simulink model "axi_filter_KCM_RC_EV"  (R2020a)
settings: Solver=VariableStepAuto  StartTime=0.0  StopTime=(height*width)/fs + (width*6)/fs + 128/fs  RelTol=1e-3
PreLoadFcn:
  | clear all;
  | 
  | fs = 100e6;
PostLoadFcn:
  | ratio = 1/6;
  | set(0,'units','pixels');
  | pixels = get(0,'screensize');
  | point1 = round(pixels(3)*ratio);
  | point2 = round(pixels(4)*ratio);
  | point3 = pixels(3)-round(pixels(3)*ratio);
  | point4 = pixels(4)-round(pixels(4)*ratio);
  | h = get_param(gcs,'handle');
  | set_param(h,'location',[point1 point2 point3 point4]);
  | pause(0.2);
  | set_param(h,'Zoomfactor','fit to view');
  | 
  | clear ratio pixels point1 point2 point3 point4 h
  | 
  | % https://uk.mathworks.com/matlabcentral/answers/358413-open-simulink-model-with-set-window-size-and-position
InitFcn:
  | height = str2num(get_param([bdroot, '/Image Properties'], 'height'));
  | width = str2num(get_param([bdroot, '/Image Properties'], 'width'));
  | I = imresize(eval(get_param([bdroot, '/Image Properties'], 'image')), [(height) (width)]);
  | I = padarray(I, [1 1], 'replicate');
  | bufferOut = uint32(double(I(:,:,1))*2^16 + double(I(:,:,3))*2^8 + double(I(:,:,2)));
  | bufferOut = reshape(bufferOut', [width+2, height+2]);
  | bufferOut = bufferOut(:);
StopFcn:
  | imtool(I);
  | imtool(uint8(reshape(bufferIn, [width, height])'));
undefined symbols (not defined in the file): AXI4, Lite
libraries: xbsIndex_r4 x114, hdlsllib x3, dspsrcs4 x2, simulink x1
(part 1 of 2)
settings Model: Creator=David Northcote  LastModifiedBy=qhb21126
settings DataIOCC: ReturnWorkspaceOutputs=off
settings DebuggingCC: ArithmeticOperatorsInVariantConditions=warning
settings SFSimCC: SimUseLocalCustomCode=off  CustomCodeUndefinedFunction=UseInterfaceOnly
settings RTWCC: RTWUseLocalCustomCode=off

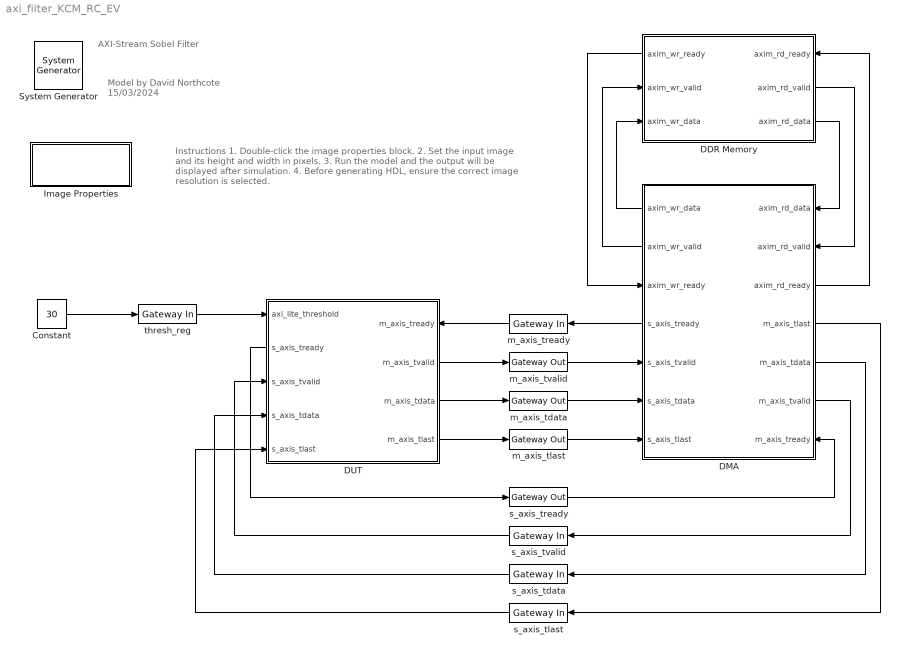
== system axi_filter_KCM_RC_EV ==
  note: Instructions
      |
      | 1. Double-click the image properties block.
      |
      | 2. Set the input image and its height and width in pixels.
      |
      | 3. Run the model and the output will be displayed after simulation.
      |
      | 4. Before generating HDL, ensure the correct image resolution is selected.
  note: Model by David Northcote
      | 15/03/2024
  note: AXI-Stream Sobel Filter
  " System Generator" : xbsIndex_r4/ System Generator  Tag=genX  xilinxfamily=zynq  part=xc7z020  speed=-1  package=clg400  synthesis_tool=Vivado  clock_wrapper=Clock Enables  directory=./netlist  proj_type=Vivado  Synth_file=Vivado Synthesis Defaults  Impl_file=Vivado Implementation Defaults  testbench=off  simulink_period=1/100e6  sysclk_period=10  dcm_input_clock_period=10  incr_netlist=off  trim_vbits=Everywhere in SubSystem  dbl_ovrd=According to Block Masks  core_generation=According to Block Masks  run_coregen=off  deprecated_control=off  eval_field=0  block_type=sysgen
  Constant : Constant  Value=30  SampleTime=-1
  DDR Memory : Subsystem  mask{bufferOut=bufferOut, dtype=uint32, outVar="bufferIn"}
      mask prompts: bufferOut "Data to be sent:"; dtype "Data type:"; outVar "Output variable name:"
      mask init:
      | dtypeStr = get_param(gcb, 'dtype');
      | outVarStr = get_param(gcb, 'outVar');
      | set_param([gcb, '/Buffer In/To Workspace'], 'VariableName', outVar)
      settings: PortSchema="{\"entries\":[{\"content\":{\"sides\":[{\"content\":{\"connectorIds\":[\"Out3\",\"In1\",\"In2\"]},\"type\":\"ConnectorPlacement.EquallySpacedRectSide\",\"uuid\":\"10820561-fcd3-42da-ac38-14c6f993f770\"},{\"content\":{\"connectorIds\":[\"In3\",\"Out1\",\"Out2\"],\"side\":\"RIGHT\"},\"type\":\"ConnectorPlacement.EquallySpacedRectSide\",\"uuid\":\"072276f7-1cf8-495f-bb0a-1bca7e8326ea\"},{\"content\":{\"connectorIds\":[],\"side\":\"TOP\"},\"type\":\"ConnectorPlacement.EquallySpacedRectSide\",\"uuid\":\"f5b81d71-f8e7-451c-95ca-ef44dafc9f7a\"}]},\"type\":\"ConnectorPlacement.EquallySpacedConnector\",\"uuid\":\"59ea238c-ea64-4381-b9ec-a479227d5ff5\"}],\"packageUris\":[\"http://schema.mathworks.com/mf0/Connector/19700101\"],\"version\":\"1.0\"}"
      mask TypeOptions dtype: uint32 | int32
      mask DialogControl DescGroupVar Prompt: DDR Memory
      mask DialogControl DescTextVar Prompt: Block simulating a DDR memory controller.
      mask DialogControl ParameterGroupVar Prompt: MM2S
      mask DialogControl Container4 Prompt: S2MM
  DMA : Subsystem  mask{N=length(bufferOut(:))}
      mask prompts: N "Length of data:"
      settings: PortSchema="{\"entries\":[{\"content\":{\"sides\":[{\"content\":{\"connectorIds\":[\"Out5\",\"Out6\",\"In1\",\"Out7\",\"In2\",\"In3\",\"In4\"]},\"type\":\"ConnectorPlacement.EquallySpacedRectSide\",\"uuid\":\"c102abcb-2e00-4fd7-85df-5b9b0b898bd0\"},{\"content\":{\"connectorIds\":[\"In5\",\"In6\",\"Out1\",\"Out2\",\"Out3\",\"Out4\",\"In7\"],\"side\":\"RIGHT\"},\"type\":\"ConnectorPlacement.EquallySpacedRectSide\",\"uuid\":\"9e178eef-1e1d-41e3-971e-2eb7c6a5387e\"},{\"content\":{\"connectorIds\":[],\"side\":\"TOP\"},\"type\":\"ConnectorPlacement.EquallySpacedRectSide\",\"uuid\":\"12cf59e0-f07a-41d8-b174-5a1eb72b1624\"},{\"content\":{\"connectorIds\":[],\"side\":\"BOTTOM\"},\"type\":\"ConnectorPlacement.EquallySpacedRectSide\",\"uuid\":\"a47cc6bb-72ec-4c9c-b625-c22428f6e2e0\"}]},\"type\":\"ConnectorPlacement.EquallySpacedConnector\",\"uuid\":\"cad21ed4-9065-49eb-a891-849a058d114a\"}],\"packageUris\":[\"http://schema.mathworks.com/mf0/Connector/19700101\"],\"version\":\"1.0\"}"
      mask DialogControl DescGroupVar Prompt: AXI DMA
      mask DialogControl DescTextVar Prompt: Block simulating an AXI DMA.
      mask DialogControl ParameterGroupVar Prompt: Main
  DUT : Subsystem
      settings: PortSchema="{\"entries\":[{\"content\":{\"sides\":[{\"content\":{\"connectorIds\":[\"In1\",\"Out4\",\"In2\",\"In3\",\"In4\"]},\"type\":\"ConnectorPlacement.EquallySpacedRectSide\",\"uuid\":\"c102abcb-2e00-4fd7-85df-5b9b0b898bd0\"},{\"content\":{\"connectorIds\":[\"In5\",\"Out1\",\"Out2\",\"Out3\"],\"side\":\"RIGHT\"},\"type\":\"ConnectorPlacement.EquallySpacedRectSide\",\"uuid\":\"9e178eef-1e1d-41e3-971e-2eb7c6a5387e\"},{\"content\":{\"connectorIds\":[],\"side\":\"TOP\"},\"type\":\"ConnectorPlacement.EquallySpacedRectSide\",\"uuid\":\"12cf59e0-f07a-41d8-b174-5a1eb72b1624\"}]},\"type\":\"ConnectorPlacement.EquallySpacedConnector\",\"uuid\":\"cad21ed4-9065-49eb-a891-849a058d114a\"}],\"packageUris\":[\"http://schema.mathworks.com/mf0/Connector/19700101\"],\"version\":\"1.0\"}"
  Image Properties : Subsystem  mask{image=imread('Louise.png'), height=317, width=313}
      mask prompts: image "Input Image:"; height "Image Height:"; width "Image Width:"
      mask init:
      | str = [width];
      mask DialogControl DescGroupVar Prompt: Image Properties
      mask DialogControl DescTextVar Prompt: Set the image and its size using the parameters below.
      mask DialogControl ParameterGroupVar Prompt: Main
      mask Display: disp('Properties')
  m_axis_tdata : xbsIndex_r4/Gateway Out  inherit_from_input=on  hdl_port=on  rows=1  columns=1  UseAsDAC=off  DACChannel='1'  interface=None  automatic_assignment=on  address_offset=hex2dec('00')  intf_name=''  intf_description=''  timing_constraint=None  locs_specified=off  LOCs={}  io_standard={}  block_type=gatewayout
  m_axis_tlast : xbsIndex_r4/Gateway Out  inherit_from_input=on  hdl_port=on  rows=1  columns=1  UseAsDAC=off  DACChannel='1'  interface=None  automatic_assignment=on  address_offset=hex2dec('00')  intf_name=''  intf_description=''  timing_constraint=None  locs_specified=off  LOCs={}  io_standard={}  block_type=gatewayout
  m_axis_tready : xbsIndex_r4/Gateway In  gui_display_data_type=Boolean  arith_type=Boolean  n_bits=16  bin_pt=14  preci_type=Single  exp_width=8  frac_width=24  rows=1  columns=1  quantization="Round  (unbiased: +/- Inf)"  overflow=Saturate  period=1/fs  UseAsADC=off  ADCChannel='1'  interface=None  automatic_assignment=on  address_offset=hex2dec('00')  intf_name=''  intf_description=''  default_value=0  timing_constraint=None  locs_specified=off  LOCs={}  io_standard={}  inherit_from_input=off  hdl_port=on  dbl_ovrd=off  block_type=gatewayin
  m_axis_tvalid : xbsIndex_r4/Gateway Out  inherit_from_input=on  hdl_port=on  rows=1  columns=1  UseAsDAC=off  DACChannel='1'  interface=None  automatic_assignment=on  address_offset=hex2dec('00')  intf_name=''  intf_description=''  timing_constraint=None  locs_specified=off  LOCs={}  io_standard={}  block_type=gatewayout
  s_axis_tdata : xbsIndex_r4/Gateway In  gui_display_data_type=Fixed-point  arith_type=Unsigned  n_bits=32  bin_pt=0  preci_type=Single  exp_width=8  frac_width=24  rows=1  columns=1  quantization="Round  (unbiased: +/- Inf)"  overflow=Saturate  period=1/fs  UseAsADC=off  ADCChannel='1'  interface=None  automatic_assignment=on  address_offset=hex2dec('00')  intf_name=''  intf_description=''  default_value=0  timing_constraint=None  locs_specified=off  LOCs={}  io_standard={}  inherit_from_input=off  hdl_port=on  dbl_ovrd=off  block_type=gatewayin
  s_axis_tlast : xbsIndex_r4/Gateway In  gui_display_data_type=Boolean  arith_type=Boolean  n_bits=16  bin_pt=14  preci_type=Single  exp_width=8  frac_width=24  rows=1  columns=1  quantization="Round  (unbiased: +/- Inf)"  overflow=Saturate  period=1/fs  UseAsADC=off  ADCChannel='1'  interface=None  automatic_assignment=on  address_offset=hex2dec('00')  intf_name=''  intf_description=''  default_value=0  timing_constraint=None  locs_specified=off  LOCs={}  io_standard={}  inherit_from_input=off  hdl_port=on  dbl_ovrd=off  block_type=gatewayin
  s_axis_tready : xbsIndex_r4/Gateway Out  inherit_from_input=on  hdl_port=on  rows=1  columns=1  UseAsDAC=off  DACChannel='1'  interface=None  automatic_assignment=on  address_offset=hex2dec('00')  intf_name=''  intf_description=''  timing_constraint=None  locs_specified=off  LOCs={}  io_standard={}  block_type=gatewayout
  s_axis_tvalid : xbsIndex_r4/Gateway In  gui_display_data_type=Boolean  arith_type=Boolean  n_bits=16  bin_pt=14  preci_type=Single  exp_width=8  frac_width=24  rows=1  columns=1  quantization="Round  (unbiased: +/- Inf)"  overflow=Saturate  period=1/fs  UseAsADC=off  ADCChannel='1'  interface=None  automatic_assignment=on  address_offset=hex2dec('00')  intf_name=''  intf_description=''  default_value=0  timing_constraint=None  locs_specified=off  LOCs={}  io_standard={}  inherit_from_input=off  hdl_port=on  dbl_ovrd=off  block_type=gatewayin
  thresh_reg : xbsIndex_r4/Gateway In  gui_display_data_type=Fixed-point  arith_type=Unsigned  n_bits=32  bin_pt=0  preci_type=Single  exp_width=8  frac_width=24  rows=1  columns=1  quantization="Round  (unbiased: +/- Inf)"  overflow=Saturate  period=1/fs  UseAsADC=off  ADCChannel='1'  interface=AXI4-Lite  automatic_assignment=on  address_offset=hex2dec('00')  intf_name=''  intf_description=''  default_value=0  timing_constraint=None  locs_specified=off  LOCs={}  io_standard={}  inherit_from_input=off  hdl_port=on  dbl_ovrd=off  block_type=gatewayin
  wires:
  s_axis_tvalid/1 -> DUT/2(s_axis_tvalid)
  s_axis_tdata/1 -> DUT/3(s_axis_tdata)
  s_axis_tlast/1 -> DUT/4(s_axis_tlast)
  m_axis_tready/1 -> DUT/5(m_axis_tready)
  DUT/4(s_axis_tready) -> s_axis_tready/1
  DUT/2(m_axis_tdata) -> m_axis_tdata/1
  DUT/1(m_axis_tvalid) -> m_axis_tvalid/1
  DUT/3(m_axis_tlast) -> m_axis_tlast/1
  s_axis_tready/1 -> DMA/7(m_axis_tready)
  DMA/4(m_axis_tvalid) -> s_axis_tvalid/1
  DMA/3(m_axis_tdata) -> s_axis_tdata/1
  DMA/2(m_axis_tlast) -> s_axis_tlast/1
  DMA/7(s_axis_tready) -> m_axis_tready/1
  m_axis_tvalid/1 -> DMA/2(s_axis_tvalid)
  m_axis_tdata/1 -> DMA/3(s_axis_tdata)
  m_axis_tlast/1 -> DMA/4(s_axis_tlast)
  DMA/1(axim_rd_ready) -> DDR Memory/3(axim_rd_ready)
  DDR Memory/1(axim_rd_valid) -> DMA/6(axim_rd_valid)
  DDR Memory/2(axim_rd_data) -> DMA/5(axim_rd_data)
  DDR Memory/3(axim_wr_ready) -> DMA/1(axim_wr_ready)
  DMA/6(axim_wr_valid) -> DDR Memory/1(axim_wr_valid)
  DMA/5(axim_wr_data) -> DDR Memory/2(axim_wr_data)
  thresh_reg/1 -> DUT/1(axi_lite_threshold)
  Constant/1 -> thresh_reg/1

== system axi_filter_KCM_RC_EV/DDR Memory ==
  axim_wr_valid : Inport
  axim_wr_data : Inport  Port=2
  axim_rd_ready : Inport  Port=3
  AXI Read Scope : Scope  NumInputPorts=3
  AXI Write Scope : Scope  NumInputPorts=3
  Buffer In : Subsystem
  Buffer Out : Subsystem
  axim_rd_valid : Outport
  axim_rd_data : Outport  Port=2
  axim_wr_ready : Outport  Port=3
  wires:
  Buffer Out/1(Valid) -> AXI Read Scope/1, axim_rd_valid/1
  Buffer Out/2(Data) -> AXI Read Scope/2, axim_rd_data/1
  axim_rd_ready/1 -> Buffer Out/Enable, AXI Read Scope/3
  axim_wr_data/1 -> AXI Write Scope/2, Buffer In/1(Data)
  Buffer In/1(Ready) -> AXI Write Scope/3, axim_wr_ready/1
  axim_wr_valid/1 -> Buffer In/Enable, AXI Write Scope/1

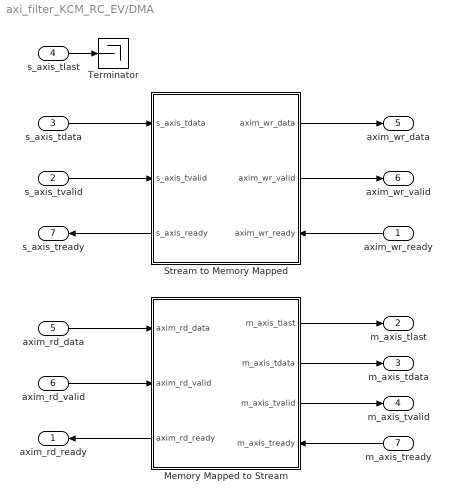
== system axi_filter_KCM_RC_EV/DMA ==
  axim_wr_ready : Inport
  s_axis_tvalid : Inport  Port=2
  s_axis_tdata : Inport  Port=3
  s_axis_tlast : Inport  Port=4
  axim_rd_data : Inport  Port=5
  axim_rd_valid : Inport  Port=6
  m_axis_tready : Inport  Port=7
  Memory Mapped to Stream : Subsystem
      settings: PortSchema="{\"entries\":[{\"content\":{\"sides\":[{\"content\":{\"connectorIds\":[\"In1\",\"In2\",\"Out4\"]},\"type\":\"ConnectorPlacement.EquallySpacedRectSide\",\"uuid\":\"10820561-fcd3-42da-ac38-14c6f993f770\"},{\"content\":{\"connectorIds\":[\"Out1\",\"Out2\",\"Out3\",\"In3\"],\"side\":\"RIGHT\"},\"type\":\"ConnectorPlacement.EquallySpacedRectSide\",\"uuid\":\"072276f7-1cf8-495f-bb0a-1bca7e8326ea\"},{\"content\":{\"connectorIds\":[],\"side\":\"TOP\"},\"type\":\"ConnectorPlacement.EquallySpacedRectSide\",\"uuid\":\"f5b81d71-f8e7-451c-95ca-ef44dafc9f7a\"}]},\"type\":\"ConnectorPlacement.EquallySpacedConnector\",\"uuid\":\"59ea238c-ea64-4381-b9ec-a479227d5ff5\"}],\"packageUris\":[\"http://schema.mathworks.com/mf0/Connector/19700101\"],\"version\":\"1.0\"}"
  Stream to Memory Mapped : Subsystem
      settings: PortSchema="{\"entries\":[{\"content\":{\"sides\":[{\"content\":{\"connectorIds\":[\"In1\",\"In2\",\"Out3\"]},\"type\":\"ConnectorPlacement.EquallySpacedRectSide\",\"uuid\":\"10820561-fcd3-42da-ac38-14c6f993f770\"},{\"content\":{\"connectorIds\":[\"Out1\",\"Out2\",\"In3\"],\"side\":\"RIGHT\"},\"type\":\"ConnectorPlacement.EquallySpacedRectSide\",\"uuid\":\"072276f7-1cf8-495f-bb0a-1bca7e8326ea\"},{\"content\":{\"connectorIds\":[],\"side\":\"TOP\"},\"type\":\"ConnectorPlacement.EquallySpacedRectSide\",\"uuid\":\"f5b81d71-f8e7-451c-95ca-ef44dafc9f7a\"}]},\"type\":\"ConnectorPlacement.EquallySpacedConnector\",\"uuid\":\"59ea238c-ea64-4381-b9ec-a479227d5ff5\"}],\"packageUris\":[\"http://schema.mathworks.com/mf0/Connector/19700101\"],\"version\":\"1.0\"}"
  Terminator : Terminator
  axim_rd_ready : Outport
  m_axis_tlast : Outport  Port=2  VectorParamsAs1DForOutWhenUnconnected=off
  m_axis_tdata : Outport  Port=3  VectorParamsAs1DForOutWhenUnconnected=off
  m_axis_tvalid : Outport  Port=4  VectorParamsAs1DForOutWhenUnconnected=off
  axim_wr_data : Outport  Port=5
  axim_wr_valid : Outport  Port=6
  s_axis_tready : Outport  Port=7  VectorParamsAs1DForOutWhenUnconnected=off
  wires:
  m_axis_tready/1 -> Memory Mapped to Stream/3(m_axis_tready)
  Memory Mapped to Stream/1(m_axis_tlast) -> m_axis_tlast/1
  Memory Mapped to Stream/2(m_axis_tdata) -> m_axis_tdata/1
  Memory Mapped to Stream/3(m_axis_tvalid) -> m_axis_tvalid/1
  s_axis_tvalid/1 -> Stream to Memory Mapped/2(s_axis_tvalid)
  s_axis_tdata/1 -> Stream to Memory Mapped/1(s_axis_tdata)
  Stream to Memory Mapped/3(s_axis_ready) -> s_axis_tready/1
  s_axis_tlast/1 -> Terminator/1
  Stream to Memory Mapped/1(axim_wr_data) -> axim_wr_data/1
  Stream to Memory Mapped/2(axim_wr_valid) -> axim_wr_valid/1
  axim_wr_ready/1 -> Stream to Memory Mapped/3(axim_wr_ready)
  Memory Mapped to Stream/4(axim_rd_ready) -> axim_rd_ready/1
  axim_rd_data/1 -> Memory Mapped to Stream/1(axim_rd_data)
  axim_rd_valid/1 -> Memory Mapped to Stream/2(axim_rd_valid)

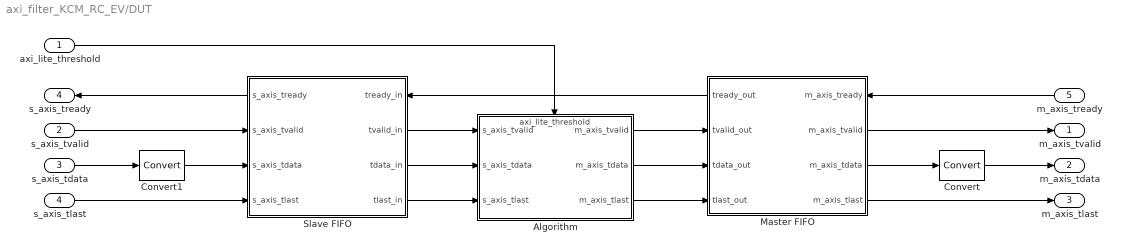
== system axi_filter_KCM_RC_EV/DUT ==
  axi_lite_threshold : Inport
  s_axis_tvalid : Inport  Port=2
  s_axis_tdata : Inport  Port=3
  s_axis_tlast : Inport  Port=4
  m_axis_tready : Inport  Port=5
  Algorithm : Subsystem
      settings: PortSchema="{\"entries\":[{\"content\":{\"sides\":[{\"content\":{\"connectorIds\":[\"In1\",\"In2\",\"In3\"]},\"type\":\"ConnectorPlacement.EquallySpacedRectSide\",\"uuid\":\"bc8f8d6b-03d4-4b1c-a4ca-076773aa8b9e\"},{\"content\":{\"connectorIds\":[\"Out1\",\"Out2\",\"Out3\"],\"side\":\"RIGHT\"},\"type\":\"ConnectorPlacement.EquallySpacedRectSide\",\"uuid\":\"0d37fd61-55f1-43d8-b642-e7957f527b3a\"},{\"content\":{\"connectorIds\":[\"In4\"],\"side\":\"TOP\"},\"type\":\"ConnectorPlacement.EquallySpacedRectSide\",\"uuid\":\"2582d54b-a3da-419d-87cd-78cc4f4daabc\"}]},\"type\":\"ConnectorPlacement.EquallySpacedConnector\",\"uuid\":\"334f8144-ee83-44bd-9d61-fffb11229a90\"}],\"packageUris\":[\"http://schema.mathworks.com/mf0/Connector/19700101\"],\"version\":\"1.0\"}"
  Convert : xbsIndex_r4/Convert  gui_display_data_type=Fixed-point  arith_type=Unsigned  n_bits=32  bin_pt=0  float_type=Single  exp_bits=8  fraction_bits=24  quantization=Truncate  overflow=Wrap  en=off  latency=0  pipeline=off  dbl_ovrd=off  block_type=convert
  Convert1 : xbsIndex_r4/Convert  gui_display_data_type=Fixed-point  arith_type=Unsigned  n_bits=24  bin_pt=0  float_type=Single  exp_bits=8  fraction_bits=24  quantization=Truncate  overflow=Wrap  en=off  latency=0  pipeline=off  dbl_ovrd=off  block_type=convert
  Master FIFO : Subsystem
      settings: PortSchema="{\"entries\":[{\"content\":{\"sides\":[{\"content\":{\"connectorIds\":[\"Out4\",\"In1\",\"In2\",\"In3\"]},\"type\":\"ConnectorPlacement.EquallySpacedRectSide\",\"uuid\":\"10820561-fcd3-42da-ac38-14c6f993f770\"},{\"content\":{\"connectorIds\":[\"In4\",\"Out1\",\"Out2\",\"Out3\"],\"side\":\"RIGHT\"},\"type\":\"ConnectorPlacement.EquallySpacedRectSide\",\"uuid\":\"072276f7-1cf8-495f-bb0a-1bca7e8326ea\"},{\"content\":{\"connectorIds\":[],\"side\":\"TOP\"},\"type\":\"ConnectorPlacement.EquallySpacedRectSide\",\"uuid\":\"f5b81d71-f8e7-451c-95ca-ef44dafc9f7a\"}]},\"type\":\"ConnectorPlacement.EquallySpacedConnector\",\"uuid\":\"59ea238c-ea64-4381-b9ec-a479227d5ff5\"}],\"packageUris\":[\"http://schema.mathworks.com/mf0/Connector/19700101\"],\"version\":\"1.0\"}"
  Slave FIFO : Subsystem
      settings: PortSchema="{\"entries\":[{\"content\":{\"sides\":[{\"content\":{\"connectorIds\":[\"Out4\",\"In1\",\"In2\",\"In3\"]},\"type\":\"ConnectorPlacement.EquallySpacedRectSide\",\"uuid\":\"10820561-fcd3-42da-ac38-14c6f993f770\"},{\"content\":{\"connectorIds\":[\"In4\",\"Out1\",\"Out2\",\"Out3\"],\"side\":\"RIGHT\"},\"type\":\"ConnectorPlacement.EquallySpacedRectSide\",\"uuid\":\"072276f7-1cf8-495f-bb0a-1bca7e8326ea\"},{\"content\":{\"connectorIds\":[],\"side\":\"TOP\"},\"type\":\"ConnectorPlacement.EquallySpacedRectSide\",\"uuid\":\"f5b81d71-f8e7-451c-95ca-ef44dafc9f7a\"}]},\"type\":\"ConnectorPlacement.EquallySpacedConnector\",\"uuid\":\"59ea238c-ea64-4381-b9ec-a479227d5ff5\"}],\"packageUris\":[\"http://schema.mathworks.com/mf0/Connector/19700101\"],\"version\":\"1.0\"}"
  m_axis_tvalid : Outport  VectorParamsAs1DForOutWhenUnconnected=off
  m_axis_tdata : Outport  Port=2  VectorParamsAs1DForOutWhenUnconnected=off
  m_axis_tlast : Outport  Port=3  VectorParamsAs1DForOutWhenUnconnected=off
  s_axis_tready : Outport  Port=4  VectorParamsAs1DForOutWhenUnconnected=off
  wires:
  Master FIFO/1(m_axis_tvalid) -> m_axis_tvalid/1
  Master FIFO/2(m_axis_tdata) -> Convert/1
  Master FIFO/3(m_axis_tlast) -> m_axis_tlast/1
  Algorithm/1(m_axis_tvalid) -> Master FIFO/1(tvalid_out)
  Algorithm/2(m_axis_tdata) -> Master FIFO/2(tdata_out)
  Algorithm/3(m_axis_tlast) -> Master FIFO/3(tlast_out)
  s_axis_tvalid/1 -> Slave FIFO/1(s_axis_tvalid)
  s_axis_tdata/1 -> Convert1/1
  s_axis_tlast/1 -> Slave FIFO/3(s_axis_tlast)
  Slave FIFO/1(tvalid_in) -> Algorithm/1(s_axis_tvalid)
  Slave FIFO/2(tdata_in) -> Algorithm/2(s_axis_tdata)
  Slave FIFO/3(tlast_in) -> Algorithm/3(s_axis_tlast)
  Slave FIFO/4(s_axis_tready) -> s_axis_tready/1
  m_axis_tready/1 -> Master FIFO/4(m_axis_tready)
  Master FIFO/4(tready_out) -> Slave FIFO/4(tready_in)
  axi_lite_threshold/1 -> Algorithm/4(axi_lite_threshold)
  Convert/1 -> m_axis_tdata/1
  Convert1/1 -> Slave FIFO/2(s_axis_tdata)

== system axi_filter_KCM_RC_EV/Image Properties ==

== system axi_filter_KCM_RC_EV/DDR Memory/Buffer In ==
  Data : Inport
  Enable : EnablePort
  Constant : Constant  OutDataTypeStr=boolean  SampleTime=-1
  To Workspace : ToWorkspace  VariableName=bufferIn  SampleTime=-1
  Ready : Outport
  wires:
  Data/1 -> To Workspace/1
  Constant/1 -> Ready/1

== system axi_filter_KCM_RC_EV/DDR Memory/Buffer Out ==
  Enable : EnablePort
  Data Type Conversion : DataTypeConversion  OutDataTypeStr=dtypeStr
  Data Type Conversion1 : DataTypeConversion  OutDataTypeStr=boolean
  Signal From Workspace : dspsrcs4/Signal From Workspace  X=bufferOut  Ts=1/fs  nsamps=1  OutputAfterFinalValue=Setting to zero  ignoreOrWarnInputAndFrameLengths=off  OutputFrames=off
  Valid Signal : dspsrcs4/Signal From Workspace  X=ones(1, length(bufferOut))  Ts=1/fs  nsamps=1  OutputAfterFinalValue=Setting to zero  ignoreOrWarnInputAndFrameLengths=off  OutputFrames=off
  Valid : Outport
  Data : Outport  Port=2
  wires:
  Signal From Workspace/1 -> Data Type Conversion/1
  Data Type Conversion/1 -> Data/1
  Valid Signal/1 -> Data Type Conversion1/1
  Data Type Conversion1/1 -> Valid/1

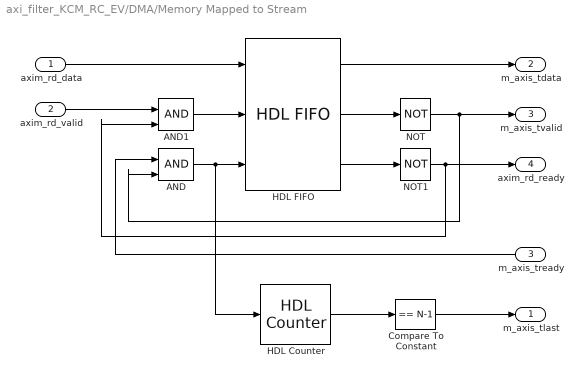
== system axi_filter_KCM_RC_EV/DMA/Memory Mapped to Stream ==
  axim_rd_data : Inport
  axim_rd_valid : Inport  Port=2
  m_axis_tready : Inport  Port=3
  AND : Logic  IconShape=distinctive  AllPortsSameDT=off  OutDataTypeStr=boolean
  AND1 : Logic  IconShape=distinctive  AllPortsSameDT=off  OutDataTypeStr=boolean
  Compare To Constant : simulink/Logic and Bit Operations/Compare To Constant  relop===  const=N-1  OutDataTypeStr=boolean
  HDL Counter : hdlsllib/Sources/HDL Counter  CountType=Count limited  CountInit=0  CountStep=1  CountMax=N-1  CountFromType=Initial value  CountFrom=0  CountResetPort=off  CountLoadPort=off  CountEnbPort=on  CountDirPort=off  CountDataType=Unsigned  CountWordLen=ceil(log2(N))  CountFracLen=0  CountSampTime=1
  HDL FIFO : hdlsllib/HDL RAMs/HDL FIFO  fifo_size=16  mode=FWFT  ratio=1  push_msg=Warning  pop_msg=Warning  show_empty=on  show_full=on  show_num=off  LabelModeActiveChoice_Mode=FWFT
      settings: SourceProductBaseCode=SL
  NOT : Logic  Operator=NOT  IconShape=distinctive  AllPortsSameDT=off  OutDataTypeStr=boolean
  NOT1 : Logic  Operator=NOT  IconShape=distinctive  AllPortsSameDT=off  OutDataTypeStr=boolean
  m_axis_tlast : Outport  VectorParamsAs1DForOutWhenUnconnected=off
  m_axis_tdata : Outport  Port=2  VectorParamsAs1DForOutWhenUnconnected=off
  m_axis_tvalid : Outport  Port=3  VectorParamsAs1DForOutWhenUnconnected=off
  axim_rd_ready : Outport  Port=4  VectorParamsAs1DForOutWhenUnconnected=off
  wires:
  NOT/1 -> m_axis_tvalid/1, AND/2
  HDL Counter/1 -> Compare To Constant/1
  m_axis_tready/1 -> AND/1
  AND/1 -> HDL Counter/1, HDL FIFO/3
  Compare To Constant/1 -> m_axis_tlast/1
  HDL FIFO/2 -> NOT/1
  AND1/1 -> HDL FIFO/2
  HDL FIFO/1 -> m_axis_tdata/1
  HDL FIFO/3 -> NOT1/1
  NOT1/1 -> AND1/2, axim_rd_ready/1
  axim_rd_valid/1 -> AND1/1
  axim_rd_data/1 -> HDL FIFO/1

== system axi_filter_KCM_RC_EV/DMA/Stream to Memory Mapped ==
  s_axis_tdata : Inport
  s_axis_tvalid : Inport  Port=2
  axim_wr_ready : Inport  Port=3
  AND : Logic  IconShape=distinctive  AllPortsSameDT=off  OutDataTypeStr=boolean
  AND1 : Logic  IconShape=distinctive  AllPortsSameDT=off  OutDataTypeStr=boolean
  HDL FIFO : hdlsllib/HDL RAMs/HDL FIFO  fifo_size=16  mode=FWFT  ratio=1  push_msg=Warning  pop_msg=Warning  show_empty=on  show_full=on  show_num=off  LabelModeActiveChoice_Mode=FWFT
      settings: SourceProductBaseCode=SL
  NOT : Logic  Operator=NOT  IconShape=distinctive  AllPortsSameDT=off  OutDataTypeStr=boolean
  NOT1 : Logic  Operator=NOT  IconShape=distinctive  AllPortsSameDT=off  OutDataTypeStr=boolean
  axim_wr_data : Outport  VectorParamsAs1DForOutWhenUnconnected=off
  axim_wr_valid : Outport  Port=2  VectorParamsAs1DForOutWhenUnconnected=off
  s_axis_ready : Outport  Port=3  VectorParamsAs1DForOutWhenUnconnected=off
  wires:
  s_axis_tvalid/1 -> AND1/1
  HDL FIFO/3 -> NOT1/1
  HDL FIFO/1 -> axim_wr_data/1
  AND1/1 -> HDL FIFO/2
  HDL FIFO/2 -> NOT/1
  AND/1 -> HDL FIFO/3
  axim_wr_ready/1 -> AND/1
  NOT/1 -> AND/2, axim_wr_valid/1
  s_axis_tdata/1 -> HDL FIFO/1
  NOT1/1 -> s_axis_ready/1, AND1/2

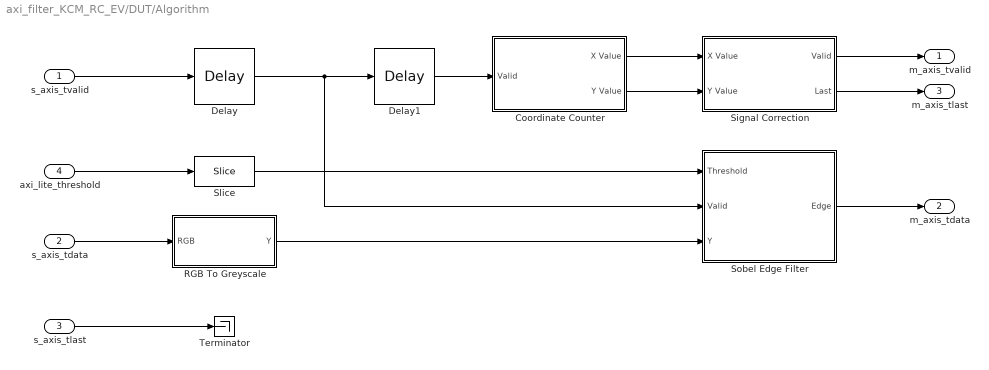
== system axi_filter_KCM_RC_EV/DUT/Algorithm ==
  s_axis_tvalid : Inport
  s_axis_tdata : Inport  Port=2
  s_axis_tlast : Inport  Port=3
  axi_lite_threshold : Inport  Port=4
  Coordinate Counter : Subsystem
  Delay : xbsIndex_r4/Delay  rst=off  infoeditControl=Selection of Reset will increase slice count due to use of real FFs and instead of SRLs  en=off  latency=3  reg_retiming=off  dbl_ovrd=off  block_type=delay
  Delay1 : xbsIndex_r4/Delay  rst=off  infoeditControl=Selection of Reset will increase slice count due to use of real FFs and instead of SRLs  en=off  latency=7  reg_retiming=off  dbl_ovrd=off  block_type=delay
  RGB To Greyscale : Subsystem
  Signal Correction : Subsystem
  Slice : xbsIndex_r4/Slice  nbits=1  boolean_output=off  mode=Two Bit Locations  bit1=7  base1=LSB of Input  bit0=0  base0=LSB of Input  dbl_ovrd=off  block_type=slice
  Sobel Edge Filter : Subsystem
  Terminator : Terminator
  m_axis_tvalid : Outport  VectorParamsAs1DForOutWhenUnconnected=off
  m_axis_tdata : Outport  Port=2  VectorParamsAs1DForOutWhenUnconnected=off
  m_axis_tlast : Outport  Port=3  VectorParamsAs1DForOutWhenUnconnected=off
  wires:
  Delay1/1 -> Coordinate Counter/1(Valid)
  Delay/1 -> Sobel Edge Filter/2(Valid), Delay1/1
  Coordinate Counter/2(Y Value) -> Signal Correction/2(Y Value)
  Coordinate Counter/1(X Value) -> Signal Correction/1(X Value)
  axi_lite_threshold/1 -> Slice/1
  s_axis_tdata/1 -> RGB To Greyscale/1(RGB)
  s_axis_tlast/1 -> Terminator/1
  s_axis_tvalid/1 -> Delay/1
  Slice/1 -> Sobel Edge Filter/1(Threshold)
  Signal Correction/2(Last) -> m_axis_tlast/1
  Signal Correction/1(Valid) -> m_axis_tvalid/1
  Sobel Edge Filter/1(Edge) -> m_axis_tdata/1
  RGB To Greyscale/1(Y) -> Sobel Edge Filter/3(Y)

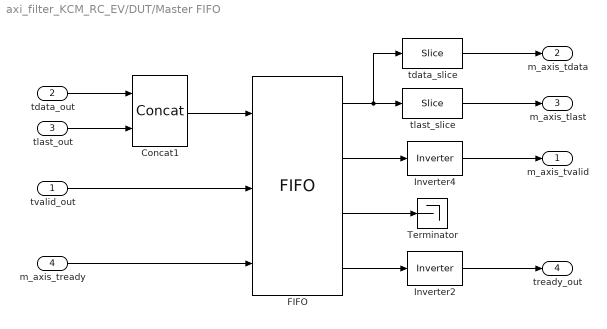
== system axi_filter_KCM_RC_EV/DUT/Master FIFO ==
  tvalid_out : Inport
  tdata_out : Inport  Port=2
  tlast_out : Inport  Port=3
  m_axis_tready : Inport  Port=4
  Concat1 : xbsIndex_r4/Concat  num_inputs=2  dbl_ovrd=off  block_type=concat
  FIFO : xbsIndex_r4/FIFO  mem_type=Block RAM  performance_options=First_Word_Fall_Through  embedded_registers=off  depth=1K  percent_nbits=1  rst=off  rst_latency=1  en=off  use_dcount=off  use_percent_full_port=off  use_almost_empty=off  almost_empty_thresh=2  use_almost_full=on  use_rd_rst_busy=off  use_wr_rst_busy=off  almost_full_thresh=1000  explicit_period=off  dbl_ovrd=off  simulation_type=fast_sim  block_type=fifo
  Inverter2 : xbsIndex_r4/Inverter  en=off  latency=0  dbl_ovrd=off  block_type=inv
  Inverter4 : xbsIndex_r4/Inverter  en=off  latency=0  dbl_ovrd=off  block_type=inv
  Terminator : Terminator
  tdata_slice : xbsIndex_r4/Slice  nbits=1  boolean_output=off  mode=Two Bit Locations  bit1=0  base1=MSB of Input  bit0=1  base0=LSB of Input  dbl_ovrd=off  block_type=slice
  tlast_slice : xbsIndex_r4/Slice  nbits=1  boolean_output=on  mode=Two Bit Locations  bit1=0  base1=LSB of Input  bit0=0  base0=LSB of Input  dbl_ovrd=off  block_type=slice
  m_axis_tvalid : Outport
  m_axis_tdata : Outport  Port=2
  m_axis_tlast : Outport  Port=3
  tready_out : Outport  Port=4
  wires:
  FIFO/4 -> Inverter2/1
  Inverter2/1 -> tready_out/1
  FIFO/2 -> Inverter4/1
  FIFO/1 -> tlast_slice/1, tdata_slice/1
  tlast_slice/1 -> m_axis_tlast/1
  tdata_slice/1 -> m_axis_tdata/1
  m_axis_tready/1 -> FIFO/3
  tvalid_out/1 -> FIFO/2
  Concat1/1 -> FIFO/1
  tdata_out/1 -> Concat1/1
  tlast_out/1 -> Concat1/2
  Inverter4/1 -> m_axis_tvalid/1
  FIFO/3 -> Terminator/1

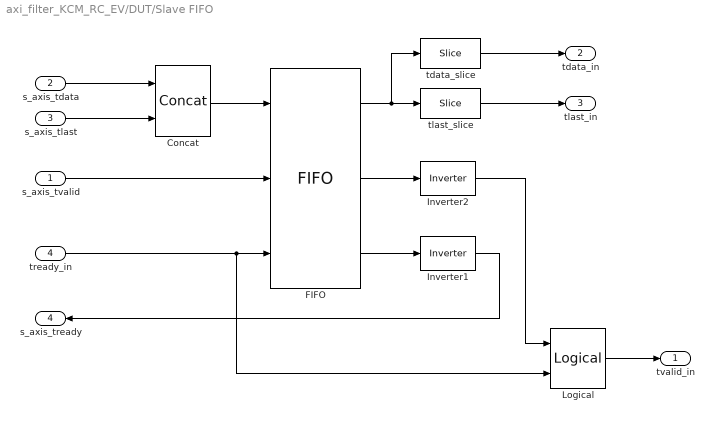
== system axi_filter_KCM_RC_EV/DUT/Slave FIFO ==
  s_axis_tvalid : Inport
  s_axis_tdata : Inport  Port=2
  s_axis_tlast : Inport  Port=3
  tready_in : Inport  Port=4
  Concat : xbsIndex_r4/Concat  num_inputs=2  dbl_ovrd=off  block_type=concat
  FIFO : xbsIndex_r4/FIFO  mem_type=Block RAM  performance_options=First_Word_Fall_Through  embedded_registers=off  depth=1K  percent_nbits=1  rst=off  rst_latency=1  en=off  use_dcount=off  use_percent_full_port=off  use_almost_empty=off  almost_empty_thresh=2  use_almost_full=off  use_rd_rst_busy=off  use_wr_rst_busy=off  almost_full_thresh=14  explicit_period=off  dbl_ovrd=off  simulation_type=fast_sim  block_type=fifo
  Inverter1 : xbsIndex_r4/Inverter  en=off  latency=0  dbl_ovrd=off  block_type=inv
  Inverter2 : xbsIndex_r4/Inverter  en=off  latency=0  dbl_ovrd=off  block_type=inv
  Logical : xbsIndex_r4/Logical  logical_function=AND  inputs=2  en=off  latency=0  precision=Full  arith_type=Unsigned  n_bits=16  bin_pt=0  align_bp=on  dbl_ovrd=off  block_type=logical
  tdata_slice : xbsIndex_r4/Slice  nbits=1  boolean_output=off  mode=Two Bit Locations  bit1=0  base1=MSB of Input  bit0=1  base0=LSB of Input  dbl_ovrd=off  block_type=slice
  tlast_slice : xbsIndex_r4/Slice  nbits=1  boolean_output=on  mode=Two Bit Locations  bit1=0  base1=LSB of Input  bit0=0  base0=LSB of Input  dbl_ovrd=off  block_type=slice
  tvalid_in : Outport
  tdata_in : Outport  Port=2
  tlast_in : Outport  Port=3
  s_axis_tready : Outport  Port=4
  wires:
  FIFO/3 -> Inverter1/1
  s_axis_tvalid/1 -> FIFO/2
  tready_in/1 -> Logical/2, FIFO/3
  Concat/1 -> FIFO/1
  s_axis_tdata/1 -> Concat/1
  s_axis_tlast/1 -> Concat/2
  FIFO/1 -> tdata_slice/1, tlast_slice/1
  tlast_slice/1 -> tlast_in/1
  tdata_slice/1 -> tdata_in/1
  Inverter1/1 -> s_axis_tready/1
  FIFO/2 -> Inverter2/1
  Inverter2/1 -> Logical/1
  Logical/1 -> tvalid_in/1

== system axi_filter_KCM_RC_EV/DUT/Algorithm/Coordinate Counter ==
  Valid : Inport
  Constant : xbsIndex_r4/Constant  const=width+1  gui_display_data_type=Fixed-point  arith_type=Unsigned  n_bits=ceil(log2(width+1))  bin_pt=0  preci_type=Single  exp_width=8  frac_width=24  explicit_period=on  period=1/100e6  equ=P=C  opselect=C  inp2=PCIN>>17  opr=+  inp1=P  carry=CIN  dbl_ovrd=off  block_type=constant
  Relational : xbsIndex_r4/Relational  mode=a=b  op_type=Bool  en=off  latency=0  dbl_ovrd=off  block_type=relational
  X Counter : xbsIndex_r4/Counter  cnt_type=Count Limited  cnt_to=width+1  operation=Up  start_count=0  cnt_by_val=1  arith_type=Unsigned  n_bits=ceil(log2(width+2))  bin_pt=0  load_pin=off  rst=off  en=on  explicit_period=off  period=1  use_behavioral_HDL=off  implementation=Fabric  dbl_ovrd=off  block_type=counter
  Y Counter : xbsIndex_r4/Counter  cnt_type=Count Limited  cnt_to=height+1  operation=Up  start_count=0  cnt_by_val=1  arith_type=Unsigned  n_bits=ceil(log2(height+2))  bin_pt=0  load_pin=off  rst=off  en=on  explicit_period=off  period=1  use_behavioral_HDL=off  implementation=Fabric  dbl_ovrd=off  block_type=counter
  X Value : Outport  VectorParamsAs1DForOutWhenUnconnected=off
  Y Value : Outport  Port=2  VectorParamsAs1DForOutWhenUnconnected=off
  wires:
  Y Counter/1 -> Y Value/1
  Valid/1 -> X Counter/1
  Relational/1 -> Y Counter/1
  X Counter/1 -> Relational/2, X Value/1
  Constant/1 -> Relational/1

== system axi_filter_KCM_RC_EV/DUT/Algorithm/RGB To Greyscale ==
  RGB : Inport
  AddSub : xbsIndex_r4/AddSub  mode=Addition  use_carryin=off  use_carryout=off  en=off  latency=1  precision=Full  arith_type=Unsigned  n_bits=16  bin_pt=14  quantization=Truncate  overflow=Wrap  use_behavioral_HDL=off  hw_selection=Fabric  pipelined=off  dbl_ovrd=off  block_type=addsub
  AddSub1 : xbsIndex_r4/AddSub  mode=Addition  use_carryin=off  use_carryout=off  en=off  latency=1  precision=User Defined  arith_type=Unsigned  n_bits=8  bin_pt=0  quantization=Truncate  overflow=Wrap  use_behavioral_HDL=off  hw_selection=Fabric  pipelined=off  dbl_ovrd=off  block_type=addsub
  Blue : xbsIndex_r4/Slice  nbits=1  boolean_output=off  mode=Two Bit Locations  bit1=15  base1=LSB of Input  bit0=8  base0=LSB of Input  dbl_ovrd=off  block_type=slice
  CMult : xbsIndex_r4/CMult  const=0.333  gui_display_data_type=Fixed-point  const_n_bits=16  const_bin_pt=15  float_type=Single  exp_bits=8  fraction_bits=24  en=off  latency=1  precision=Full  arith_type="Signed  (2's comp)"  n_bits=16  bin_pt=14  quantization=Truncate  overflow=Wrap  use_behavioral_HDL=off  mem_type=Distributed RAM  pipeline=off  dbl_ovrd=off  block_type=cmult
  CMult1 : xbsIndex_r4/CMult  const=0.333  gui_display_data_type=Fixed-point  const_n_bits=16  const_bin_pt=15  float_type=Single  exp_bits=8  fraction_bits=24  en=off  latency=1  precision=Full  arith_type="Signed  (2's comp)"  n_bits=16  bin_pt=14  quantization=Truncate  overflow=Wrap  use_behavioral_HDL=off  mem_type=Distributed RAM  pipeline=off  dbl_ovrd=off  block_type=cmult
  CMult2 : xbsIndex_r4/CMult  const=0.333  gui_display_data_type=Fixed-point  const_n_bits=16  const_bin_pt=15  float_type=Single  exp_bits=8  fraction_bits=24  en=off  latency=1  precision=Full  arith_type="Signed  (2's comp)"  n_bits=16  bin_pt=14  quantization=Truncate  overflow=Wrap  use_behavioral_HDL=off  mem_type=Distributed RAM  pipeline=off  dbl_ovrd=off  block_type=cmult
  Green : xbsIndex_r4/Slice  nbits=1  boolean_output=off  mode=Two Bit Locations  bit1=7  base1=LSB of Input  bit0=0  base0=LSB of Input  dbl_ovrd=off  block_type=slice
  Red : xbsIndex_r4/Slice  nbits=1  boolean_output=off  mode=Two Bit Locations  bit1=23  base1=LSB of Input  bit0=16  base0=LSB of Input  dbl_ovrd=off  block_type=slice
  Register : xbsIndex_r4/Register  init=0  rst=off  en=off  dbl_ovrd=off  block_type=register
  Y : Outport  VectorParamsAs1DForOutWhenUnconnected=off
  wires:
  AddSub/1 -> AddSub1/1
  Register/1 -> AddSub1/2
  CMult1/1 -> Register/1
  CMult2/1 -> AddSub/2
  CMult/1 -> AddSub/1
  RGB/1 -> Red/1, Blue/1, Green/1
  Blue/1 -> CMult2/1
  Red/1 -> CMult/1
  Green/1 -> CMult1/1
  AddSub1/1 -> Y/1

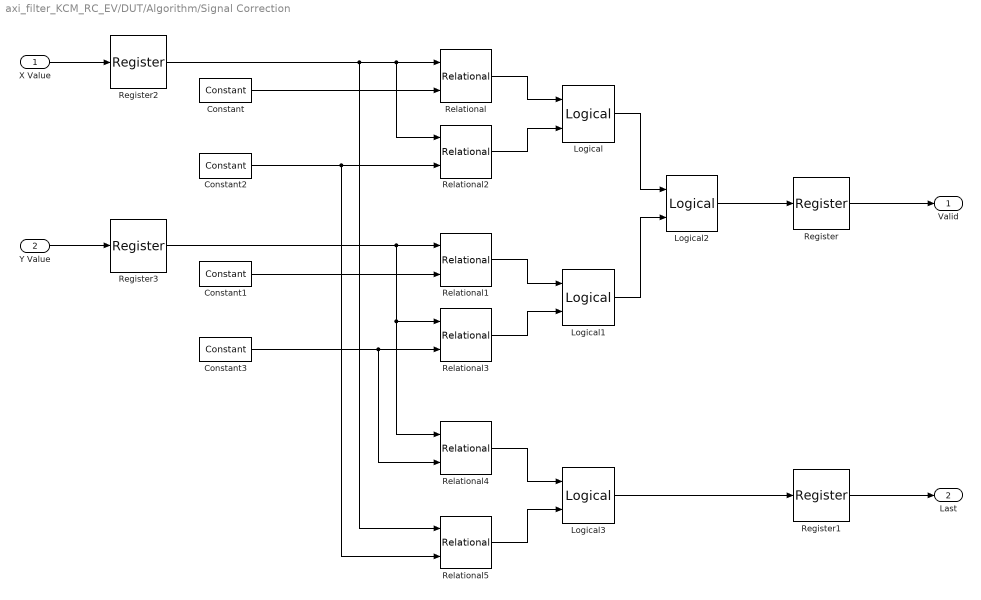
== system axi_filter_KCM_RC_EV/DUT/Algorithm/Signal Correction ==
  X Value : Inport
  Y Value : Inport  Port=2
  Constant : xbsIndex_r4/Constant  const=1  gui_display_data_type=Fixed-point  arith_type=Unsigned  n_bits=ceil(log2(width+1))  bin_pt=0  preci_type=Single  exp_width=8  frac_width=24  explicit_period=on  period=1/100e6  equ=P=C  opselect=C  inp2=PCIN>>17  opr=+  inp1=P  carry=CIN  dbl_ovrd=off  block_type=constant
  Constant1 : xbsIndex_r4/Constant  const=1  gui_display_data_type=Fixed-point  arith_type=Unsigned  n_bits=ceil(log2(height+1))  bin_pt=0  preci_type=Single  exp_width=8  frac_width=24  explicit_period=on  period=1/100e6  equ=P=C  opselect=C  inp2=PCIN>>17  opr=+  inp1=P  carry=CIN  dbl_ovrd=off  block_type=constant
  Constant2 : xbsIndex_r4/Constant  const=width  gui_display_data_type=Fixed-point  arith_type=Unsigned  n_bits=ceil(log2(width+1))  bin_pt=0  preci_type=Single  exp_width=8  frac_width=24  explicit_period=on  period=1/100e6  equ=P=C  opselect=C  inp2=PCIN>>17  opr=+  inp1=P  carry=CIN  dbl_ovrd=off  block_type=constant
  Constant3 : xbsIndex_r4/Constant  const=height  gui_display_data_type=Fixed-point  arith_type=Unsigned  n_bits=ceil(log2(height+1))  bin_pt=0  preci_type=Single  exp_width=8  frac_width=24  explicit_period=on  period=1/100e6  equ=P=C  opselect=C  inp2=PCIN>>17  opr=+  inp1=P  carry=CIN  dbl_ovrd=off  block_type=constant
  Logical{,1..3} (4 alike) : xbsIndex_r4/Logical  logical_function=AND  inputs=2  en=off  latency=0  precision=Full  arith_type=Unsigned  n_bits=16  bin_pt=0  align_bp=on  dbl_ovrd=off  block_type=logical
  Register{,1..3} (4 alike) : xbsIndex_r4/Register  init=0  rst=off  en=off  dbl_ovrd=off  block_type=register
  Relational : xbsIndex_r4/Relational  mode=a>=b  op_type=Bool  en=off  latency=0  dbl_ovrd=off  block_type=relational
  Relational1 : xbsIndex_r4/Relational  mode=a>=b  op_type=Bool  en=off  latency=0  dbl_ovrd=off  block_type=relational
  Relational2 : xbsIndex_r4/Relational  mode=a<=b  op_type=Bool  en=off  latency=0  dbl_ovrd=off  block_type=relational
  Relational3 : xbsIndex_r4/Relational  mode=a<=b  op_type=Bool  en=off  latency=0  dbl_ovrd=off  block_type=relational
  Relational4 : xbsIndex_r4/Relational  mode=a=b  op_type=Bool  en=off  latency=0  dbl_ovrd=off  block_type=relational
  Relational5 : xbsIndex_r4/Relational  mode=a=b  op_type=Bool  en=off  latency=0  dbl_ovrd=off  block_type=relational
  Valid : Outport  VectorParamsAs1DForOutWhenUnconnected=off
  Last : Outport  Port=2  VectorParamsAs1DForOutWhenUnconnected=off
  wires:
  Register3/1 -> Relational1/1, Relational3/1, Relational4/1
  Register2/1 -> Relational2/1, Relational/1, Relational5/1
  Register1/1 -> Last/1
  Logical3/1 -> Register1/1
  Relational5/1 -> Logical3/2
  Relational4/1 -> Logical3/1
  Register/1 -> Valid/1
  Logical2/1 -> Register/1
  Logical1/1 -> Logical2/2
  Logical/1 -> Logical2/1
  Relational3/1 -> Logical1/2
  Relational1/1 -> Logical1/1
  Constant3/1 -> Relational3/2, Relational4/2
  Y Value/1 -> Register3/1
  Relational/1 -> Logical/1
  Relational2/1 -> Logical/2
  X Value/1 -> Register2/1
  Constant2/1 -> Relational2/2, Relational5/2
  Constant1/1 -> Relational1/2
  Constant/1 -> Relational/2

== system axi_filter_KCM_RC_EV/DUT/Algorithm/Sobel Edge Filter ==
  Threshold : Inport
  Valid : Inport  Port=2
  Y : Inport  Port=3
  Filter Function : Subsystem
  Filter Window : Subsystem
  Gradient Approximation : Subsystem
  Thresholding : Subsystem
  Edge : Outport  VectorParamsAs1DForOutWhenUnconnected=off
  wires:
  Valid/1 -> Filter Window/2(Valid)
  Threshold/1 -> Thresholding/1(Threshold)
  Gradient Approximation/1(Gmag) -> Thresholding/2(Gmag)
  Y/1 -> Filter Window/1(Pixel)
  Filter Window/5(w11) -> Filter Function/5(w11)
  Filter Window/3(w02) -> Filter Function/3(w02)
  Filter Window/9(w22) -> Filter Function/9(w22)
  Filter Window/2(w01) -> Filter Function/2(w01)
  Filter Window/7(w20) -> Filter Function/7(w20)
  Filter Window/4(w10) -> Filter Function/4(w10)
  Filter Window/6(w12) -> Filter Function/6(w12)
  Filter Window/1(w00) -> Filter Function/1(w00)
  Filter Window/8(w21) -> Filter Function/8(w21)
  Thresholding/1(Edge) -> Edge/1
  Filter Function/1(Gx) -> Gradient Approximation/1(Gx)
  Filter Function/2(Gy) -> Gradient Approximation/2(Gy)

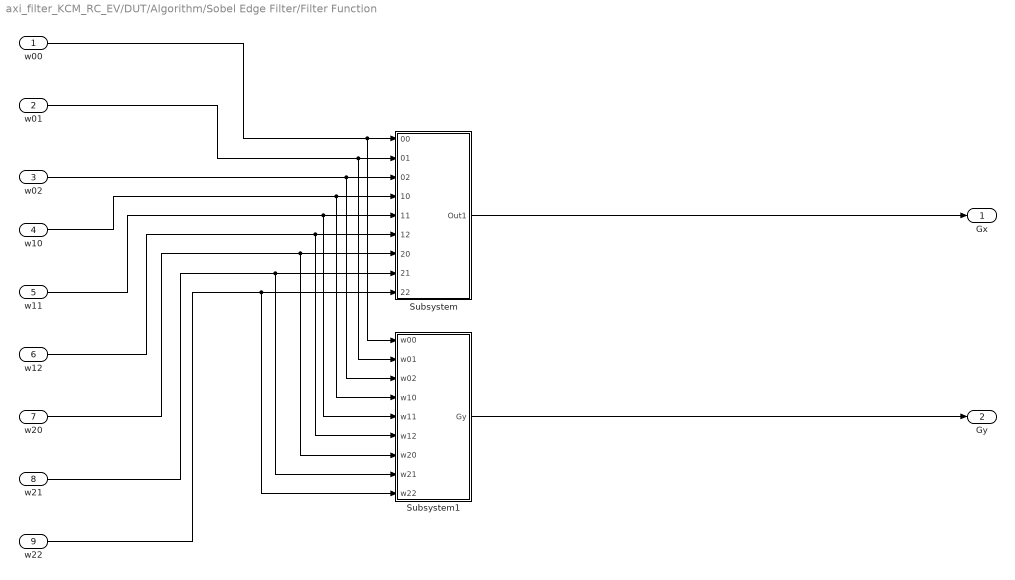
== system axi_filter_KCM_RC_EV/DUT/Algorithm/Sobel Edge Filter/Filter Function ==
  w00 : Inport
  w01 : Inport  Port=2
  w02 : Inport  Port=3
  w10 : Inport  Port=4
  w11 : Inport  Port=5
  w12 : Inport  Port=6
  w20 : Inport  Port=7
  w21 : Inport  Port=8
  w22 : Inport  Port=9
  Subsystem : Subsystem
  Subsystem1 : Subsystem
  Gx : Outport  VectorParamsAs1DForOutWhenUnconnected=off
  Gy : Outport  Port=2  VectorParamsAs1DForOutWhenUnconnected=off
  wires:
  w00/1 -> Subsystem1/1(w00), Subsystem/1(00)
  w01/1 -> Subsystem1/2(w01), Subsystem/2(01)
  w02/1 -> Subsystem1/3(w02), Subsystem/3(02)
  w10/1 -> Subsystem1/4(w10), Subsystem/4(10)
  w11/1 -> Subsystem1/5(w11), Subsystem/5(11)
  w12/1 -> Subsystem1/6(w12), Subsystem/6(12)
  w21/1 -> Subsystem1/8(w21), Subsystem/8(21)
  w22/1 -> Subsystem1/9(w22), Subsystem/9(22)
  Subsystem/1(Out1) -> Gx/1
  Subsystem1/1(Gy) -> Gy/1
  w20/1 -> Subsystem1/7(w20), Subsystem/7(20)

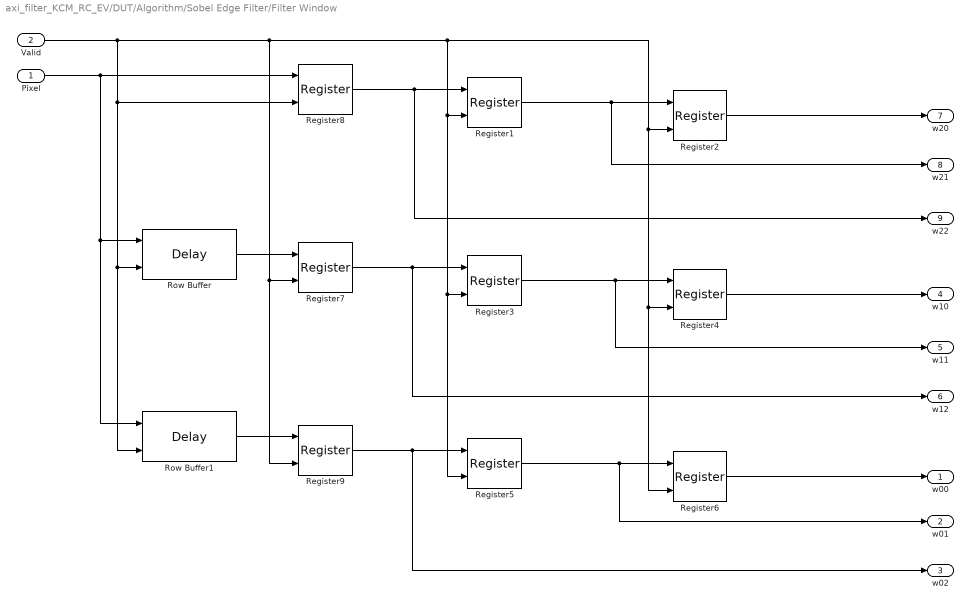
== system axi_filter_KCM_RC_EV/DUT/Algorithm/Sobel Edge Filter/Filter Window ==
  Pixel : Inport
  Valid : Inport  Port=2
  Register{1..9} (9 alike) : xbsIndex_r4/Register  init=0  rst=off  en=on  dbl_ovrd=off  block_type=register
  Row Buffer : xbsIndex_r4/Delay  rst=off  infoeditControl=Selection of Reset will increase slice count due to use of real FFs and instead of SRLs  en=on  latency=width+2  reg_retiming=off  dbl_ovrd=off  block_type=delay
  Row Buffer1 : xbsIndex_r4/Delay  rst=off  infoeditControl=Selection of Reset will increase slice count due to use of real FFs and instead of SRLs  en=on  latency=width+2  reg_retiming=off  dbl_ovrd=off  block_type=delay
  w00 : Outport  VectorParamsAs1DForOutWhenUnconnected=off
  w01 : Outport  Port=2  VectorParamsAs1DForOutWhenUnconnected=off
  w02 : Outport  Port=3  VectorParamsAs1DForOutWhenUnconnected=off
  w10 : Outport  Port=4  VectorParamsAs1DForOutWhenUnconnected=off
  w11 : Outport  Port=5  VectorParamsAs1DForOutWhenUnconnected=off
  w12 : Outport  Port=6  VectorParamsAs1DForOutWhenUnconnected=off
  w20 : Outport  Port=7  VectorParamsAs1DForOutWhenUnconnected=off
  w21 : Outport  Port=8  VectorParamsAs1DForOutWhenUnconnected=off
  w22 : Outport  Port=9  VectorParamsAs1DForOutWhenUnconnected=off
  wires:
  Valid/1 -> Register2/2, Register4/2, Register6/2, Register1/2, Register3/2, Register5/2, Register7/2, Register9/2, Register8/2, Row Buffer/2, Row Buffer1/2
  Register9/1 -> Register5/1, w02/1
  Register8/1 -> w22/1, Register1/1
  Register7/1 -> Register3/1, w12/1
  Register4/1 -> w10/1
  Register6/1 -> w00/1
  Register3/1 -> w11/1, Register4/1
  Register2/1 -> w20/1
  Row Buffer1/1 -> Register9/1
  Register5/1 -> w01/1, Register6/1
  Register1/1 -> w21/1, Register2/1
  Pixel/1 -> Register8/1, Row Buffer/1, Row Buffer1/1
  Row Buffer/1 -> Register7/1

== system axi_filter_KCM_RC_EV/DUT/Algorithm/Sobel Edge Filter/Gradient Approximation ==
  Gx : Inport
  Gy : Inport  Port=2
  Absolute : xbsIndex_r4/Absolute  precision=Full  arith_type=Unsigned  n_bits=16  bin_pt=14  quantization=Truncate  overflow=Wrap  en=off  latency=1  dbl_ovrd=off  block_type=abs
  Absolute1 : xbsIndex_r4/Absolute  precision=Full  arith_type=Unsigned  n_bits=16  bin_pt=14  quantization=Truncate  overflow=Wrap  en=off  latency=1  dbl_ovrd=off  block_type=abs
  AddSub : xbsIndex_r4/AddSub  mode=Addition  use_carryin=off  use_carryout=off  en=off  latency=1  precision=Full  arith_type=Unsigned  n_bits=16  bin_pt=14  quantization=Truncate  overflow=Wrap  use_behavioral_HDL=off  hw_selection=Fabric  pipelined=off  dbl_ovrd=off  block_type=addsub
  Shift : xbsIndex_r4/Shift  shift_dir=Right  shift_bits=2  en=off  latency=1  precision=User Defined  arith_type=Unsigned  n_bits=8  bin_pt=0  quantization=Truncate  overflow=Wrap  dbl_ovrd=off  block_type=shift
  Gmag : Outport  VectorParamsAs1DForOutWhenUnconnected=off
  wires:
  Shift/1 -> Gmag/1
  AddSub/1 -> Shift/1
  Absolute1/1 -> AddSub/2
  Absolute/1 -> AddSub/1
  Gy/1 -> Absolute1/1
  Gx/1 -> Absolute/1

== system axi_filter_KCM_RC_EV/DUT/Algorithm/Sobel Edge Filter/Thresholding ==
  Threshold : Inport
  Gmag : Inport  Port=2
  Constant : xbsIndex_r4/Constant  const=255  gui_display_data_type=Fixed-point  arith_type=Unsigned  n_bits=8  bin_pt=0  preci_type=Single  exp_width=8  frac_width=24  explicit_period=on  period=1/100e6  equ=P=C  opselect=C  inp2=PCIN>>17  opr=+  inp1=P  carry=CIN  dbl_ovrd=off  block_type=constant
  Constant1 : xbsIndex_r4/Constant  const=0  gui_display_data_type=Fixed-point  arith_type=Unsigned  n_bits=8  bin_pt=0  preci_type=Single  exp_width=8  frac_width=24  explicit_period=on  period=1/100e6  equ=P=C  opselect=C  inp2=PCIN>>17  opr=+  inp1=P  carry=CIN  dbl_ovrd=off  block_type=constant
  Mux : xbsIndex_r4/Mux  inputs=2  en=off  latency=1  precision=Full  arith_type=Unsigned  n_bits=16  bin_pt=14  quantization=Truncate  overflow=Wrap  dbl_ovrd=off  block_type=mux
  Relational : xbsIndex_r4/Relational  mode=a>=b  op_type=Bool  en=off  latency=0  dbl_ovrd=off  block_type=relational
  Edge : Outport  VectorParamsAs1DForOutWhenUnconnected=off
  wires:
  Threshold/1 -> Relational/2
  Relational/1 -> Mux/1
  Constant/1 -> Mux/3
  Constant1/1 -> Mux/2
  Gmag/1 -> Relational/1
  Mux/1 -> Edge/1

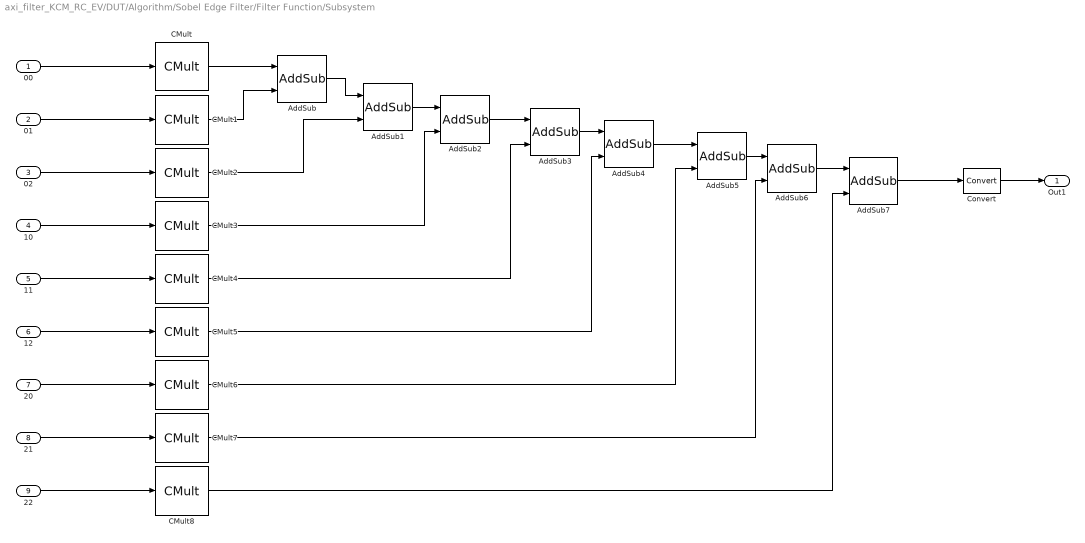
== system axi_filter_KCM_RC_EV/DUT/Algorithm/Sobel Edge Filter/Filter Function/Subsystem ==
  00 : Inport
  01 : Inport  Port=2
  02 : Inport  Port=3
  10 : Inport  Port=4
  11 : Inport  Port=5
  12 : Inport  Port=6
  20 : Inport  Port=7
  21 : Inport  Port=8
  22 : Inport  Port=9
  AddSub{,1..7} (8 alike) : xbsIndex_r4/AddSub  mode=Addition  use_carryin=off  use_carryout=off  en=off  latency=1  precision=Full  arith_type=Unsigned  n_bits=16  bin_pt=14  quantization=Truncate  overflow=Wrap  use_behavioral_HDL=off  hw_selection=Fabric  pipelined=off  dbl_ovrd=off  block_type=addsub
  CMult : xbsIndex_r4/CMult  const=1  gui_display_data_type=Fixed-point  const_n_bits=4  const_bin_pt=0  float_type=Single  exp_bits=8  fraction_bits=24  en=off  latency=1  precision=Full  arith_type="Signed  (2's comp)"  n_bits=16  bin_pt=14  quantization=Truncate  overflow=Wrap  use_behavioral_HDL=off  mem_type=Distributed RAM  pipeline=off  dbl_ovrd=off  block_type=cmult
  CMult1 : xbsIndex_r4/CMult  const=0  gui_display_data_type=Fixed-point  const_n_bits=4  const_bin_pt=0  float_type=Single  exp_bits=8  fraction_bits=24  en=off  latency=1  precision=Full  arith_type="Signed  (2's comp)"  n_bits=16  bin_pt=14  quantization=Truncate  overflow=Wrap  use_behavioral_HDL=off  mem_type=Distributed RAM  pipeline=off  dbl_ovrd=off  block_type=cmult
  CMult2 : xbsIndex_r4/CMult  const=-1  gui_display_data_type=Fixed-point  const_n_bits=4  const_bin_pt=0  float_type=Single  exp_bits=8  fraction_bits=24  en=off  latency=1  precision=Full  arith_type="Signed  (2's comp)"  n_bits=16  bin_pt=14  quantization=Truncate  overflow=Wrap  use_behavioral_HDL=off  mem_type=Distributed RAM  pipeline=off  dbl_ovrd=off  block_type=cmult
  CMult3 : xbsIndex_r4/CMult  const=2  gui_display_data_type=Fixed-point  const_n_bits=4  const_bin_pt=0  float_type=Single  exp_bits=8  fraction_bits=24  en=off  latency=1  precision=Full  arith_type="Signed  (2's comp)"  n_bits=16  bin_pt=14  quantization=Truncate  overflow=Wrap  use_behavioral_HDL=off  mem_type=Distributed RAM  pipeline=off  dbl_ovrd=off  block_type=cmult
  CMult4 : xbsIndex_r4/CMult  const=0  gui_display_data_type=Fixed-point  const_n_bits=4  const_bin_pt=0  float_type=Single  exp_bits=8  fraction_bits=24  en=off  latency=1  precision=Full  arith_type="Signed  (2's comp)"  n_bits=16  bin_pt=14  quantization=Truncate  overflow=Wrap  use_behavioral_HDL=off  mem_type=Distributed RAM  pipeline=off  dbl_ovrd=off  block_type=cmult
  CMult5 : xbsIndex_r4/CMult  const=-2  gui_display_data_type=Fixed-point  const_n_bits=4  const_bin_pt=0  float_type=Single  exp_bits=8  fraction_bits=24  en=off  latency=1  precision=Full  arith_type="Signed  (2's comp)"  n_bits=16  bin_pt=14  quantization=Truncate  overflow=Wrap  use_behavioral_HDL=off  mem_type=Distributed RAM  pipeline=off  dbl_ovrd=off  block_type=cmult
  CMult6 : xbsIndex_r4/CMult  const=1  gui_display_data_type=Fixed-point  const_n_bits=4  const_bin_pt=0  float_type=Single  exp_bits=8  fraction_bits=24  en=off  latency=1  precision=Full  arith_type="Signed  (2's comp)"  n_bits=16  bin_pt=14  quantization=Truncate  overflow=Wrap  use_behavioral_HDL=off  mem_type=Distributed RAM  pipeline=off  dbl_ovrd=off  block_type=cmult
  CMult7 : xbsIndex_r4/CMult  const=0  gui_display_data_type=Fixed-point  const_n_bits=4  const_bin_pt=0  float_type=Single  exp_bits=8  fraction_bits=24  en=off  latency=1  precision=Full  arith_type="Signed  (2's comp)"  n_bits=16  bin_pt=14  quantization=Truncate  overflow=Wrap  use_behavioral_HDL=off  mem_type=Distributed RAM  pipeline=off  dbl_ovrd=off  block_type=cmult
  CMult8 : xbsIndex_r4/CMult  const=-1  gui_display_data_type=Fixed-point  const_n_bits=4  const_bin_pt=0  float_type=Single  exp_bits=8  fraction_bits=24  en=off  latency=1  precision=Full  arith_type="Signed  (2's comp)"  n_bits=16  bin_pt=14  quantization=Truncate  overflow=Wrap  use_behavioral_HDL=off  mem_type=Distributed RAM  pipeline=off  dbl_ovrd=off  block_type=cmult
  Convert : xbsIndex_r4/Convert  gui_display_data_type=Fixed-point  arith_type=Unsigned  n_bits=24  bin_pt=0  float_type=Single  exp_bits=8  fraction_bits=24  quantization=Truncate  overflow=Saturate  en=off  latency=1  pipeline=off  dbl_ovrd=off  block_type=convert
  Out1 : Outport
  wires:
  AddSub2/1 -> AddSub3/1
  AddSub3/1 -> AddSub4/1
  CMult/1 -> AddSub/1
  CMult6/1 -> AddSub5/2
  AddSub1/1 -> AddSub2/1
  20/1 -> CMult6/1
  CMult2/1 -> AddSub1/2
  AddSub6/1 -> AddSub7/1
  CMult7/1 -> AddSub6/2
  CMult5/1 -> AddSub4/2
  00/1 -> CMult/1
  AddSub5/1 -> AddSub6/1
  CMult4/1 -> AddSub3/2
  CMult3/1 -> AddSub2/2
  CMult1/1 -> AddSub/2
  CMult8/1 -> AddSub7/2
  AddSub4/1 -> AddSub5/1
  02/1 -> CMult2/1
  01/1 -> CMult1/1
  AddSub/1 -> AddSub1/1
  10/1 -> CMult3/1
  22/1 -> CMult8/1
  AddSub7/1 -> Convert/1
  21/1 -> CMult7/1
  12/1 -> CMult5/1
  11/1 -> CMult4/1
  Convert/1 -> Out1/1
